simulink model "cars1"  (Simulink 7.6)
settings: Solver=ode45  StartTime=0.0  StopTime=60  RelTol=1e-3
libraries: simulink x2
settings Model: Creator=Bogdy  LastModifiedBy=Bogdy
settings OptimizationCC: BlockReduction=off  BooleanDataType=off
settings DebuggingCC: SaveWithParameterizedLinksMsg=none  SignalResolutionControl=TryResolveAllWithWarning  SolverPrmCheckMsg=none  MultiTaskDSMMsg=warning  MultiTaskCondExecSysMsg=none  StrictBusMsg=None
settings HardwareCC: TargetUnknown=on
settings RTWCC: IncludeERTFirstTime=on

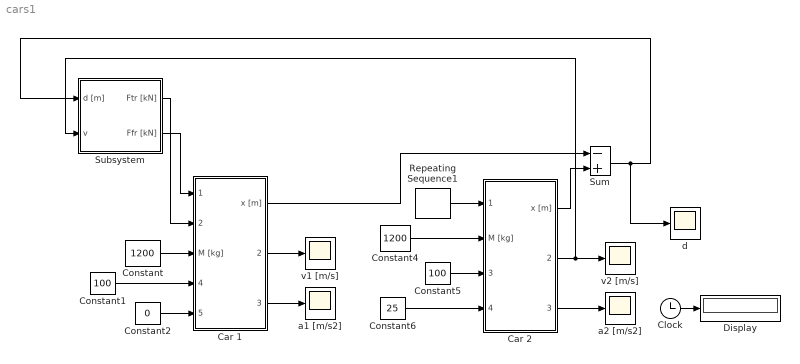
== system cars1 ==
  Car 1 : Subsystem
  Car 2 : Subsystem
  Clock : Clock
      settings: Decimation=10
  Constant : Constant  Value=1200
  Constant1 : Constant  Value=100
  Constant2 : Constant  Value=0
  Constant4 : Constant  Value=1200
  Constant5 : Constant  Value=100
  Constant6 : Constant  Value=25
  Display : Display
  Repeating Sequence1 : simulink/Sources/Repeating Sequence  SystemSampleTime=-1  rep_seq_t=[0 1 5 10 20 30 40 50 59 60]  rep_seq_y=[1 4 4 0 -2 -3 1 2 -1 1]
  Subsystem : Subsystem
  Sum : Sum  Inputs=-+  SaturateOnIntegerOverflow=on  InputSameDT=on  OutDataTypeStr=Inherit: Same as first input
  a1 [m/s2] : Scope
      settings: TimeRange=70  YMin=-4  YMax=4  SaveName=ScopeData2
  a2 [m/s2] : Scope
      settings: SaveName=ScopeData3
  d : Scope
      settings: TimeRange=60  YMin=0  YMax=550
  v1 [m/s] : Scope
  v2 [m/s] : Scope
      settings: YMin=0  YMax=550  SaveName=ScopeData4
  wires:
  Car 1/2(v [km/h]) -> v1 [m/s]/1
  Car 1/3(a [m/s2]) -> a1 [m/s2]/1
  Constant/1 -> Car 1/3(M [kg])
  Constant1/1 -> Car 1/4(V0 [km/h])
  Constant2/1 -> Car 1/5(X0 [m])
  Car 2/2(v [km/h]) -> v2 [m/s]/1, Subsystem/2(v)
  Car 2/3(a [m/s2]) -> a2 [m/s2]/1
  Constant4/1 -> Car 2/2(M [kg])
  Constant5/1 -> Car 2/3(V0 [km/h])
  Constant6/1 -> Car 2/4(X0 [m])
  Repeating Sequence1/1 -> Car 2/1(Ftr [kN])
  Sum/1 -> Subsystem/1(d [m]), d/1
  Clock/1 -> Display/1
  Subsystem/1(Ftr [kN]) -> Car 1/2(Ffr [kN])
  Subsystem/2(Ffr [kN]) -> Car 1/1(Ftr [kN])
  Car 2/1(x [m]) -> Sum/2
  Car 1/1(x [m]) -> Sum/1

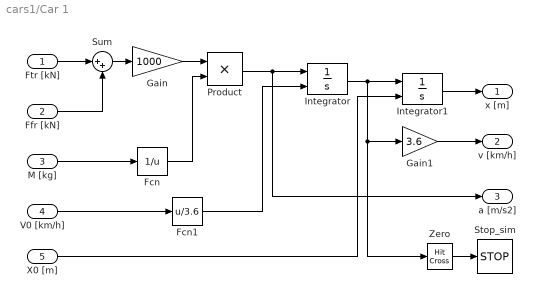
== system cars1/Car 1 ==
  Ftr [kN] : Inport
  Ffr [kN] : Inport  Port=2
  M [kg] : Inport  Port=3
  V0 [km/h] : Inport  Port=4
  X0 [m] : Inport  Port=5
  Fcn : Fcn  Expr=1/u
  Fcn1 : Fcn  Expr=u/3.6
  Gain : Gain  Gain=1000  SaturateOnIntegerOverflow=on  OutDataTypeStr=Inherit: Same as input  ParamDataTypeStr=Inherit: Same as input
  Gain1 : Gain  Gain=3.6  SaturateOnIntegerOverflow=on  OutDataTypeStr=Inherit: Same as input  ParamDataTypeStr=Inherit: Same as input
  Integrator : Integrator  InitialConditionSource=external
  Integrator1 : Integrator  InitialConditionSource=external
  Product : Product  SaturateOnIntegerOverflow=on  RndMeth=Zero  InputSameDT=on  OutDataTypeStr=Inherit: Same as first input
  Stop_sim : Stop
  Sum : Sum  Inputs=|++  SaturateOnIntegerOverflow=on  InputSameDT=on  OutDataTypeStr=Inherit: Same as first input
  Zero : HitCross  HitCrossingOffset=1  HitCrossingDirection=falling
  x [m] : Outport
  v [km/h] : Outport  Port=2
  a [m/s2] : Outport  Port=3
  wires:
  Ffr [kN]/1 -> Sum/2
  M [kg]/1 -> Fcn/1
  Sum/1 -> Gain/1
  Fcn/1 -> Product/2
  Product/1 -> Integrator/1, a [m/s2]/1
  V0 [km/h]/1 -> Fcn1/1
  Integrator/1 -> Integrator1/1, Gain1/1, Zero/1
  X0 [m]/1 -> Integrator1/2
  Integrator1/1 -> x [m]/1
  Fcn1/1 -> Integrator/2
  Gain1/1 -> v [km/h]/1
  Zero/1 -> Stop_sim/1
  Ftr [kN]/1 -> Sum/1
  Gain/1 -> Product/1

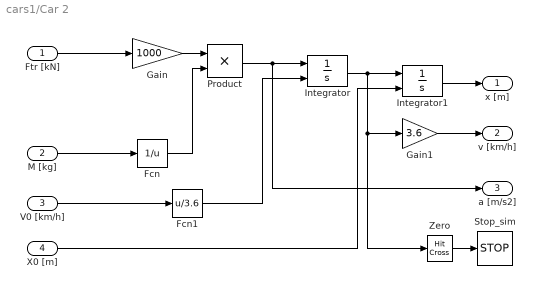
== system cars1/Car 2 ==
  Ftr [kN] : Inport
  M [kg] : Inport  Port=2
  V0 [km/h] : Inport  Port=3
  X0 [m] : Inport  Port=4
  Fcn : Fcn  Expr=1/u
  Fcn1 : Fcn  Expr=u/3.6
  Gain : Gain  Gain=1000  SaturateOnIntegerOverflow=on  OutDataTypeStr=Inherit: Same as input  ParamDataTypeStr=Inherit: Same as input
  Gain1 : Gain  Gain=3.6  SaturateOnIntegerOverflow=on  OutDataTypeStr=Inherit: Same as input  ParamDataTypeStr=Inherit: Same as input
  Integrator : Integrator  InitialConditionSource=external
  Integrator1 : Integrator  InitialConditionSource=external
  Product : Product  SaturateOnIntegerOverflow=on  RndMeth=Zero  InputSameDT=on  OutDataTypeStr=Inherit: Same as first input
  Stop_sim : Stop
  Zero : HitCross  HitCrossingOffset=1  HitCrossingDirection=falling
  x [m] : Outport
  v [km/h] : Outport  Port=2
  a [m/s2] : Outport  Port=3
  wires:
  M [kg]/1 -> Fcn/1
  Fcn/1 -> Product/2
  Product/1 -> Integrator/1, a [m/s2]/1
  V0 [km/h]/1 -> Fcn1/1
  Integrator/1 -> Integrator1/1, Gain1/1, Zero/1
  X0 [m]/1 -> Integrator1/2
  Integrator1/1 -> x [m]/1
  Fcn1/1 -> Integrator/2
  Gain1/1 -> v [km/h]/1
  Zero/1 -> Stop_sim/1
  Ftr [kN]/1 -> Gain/1
  Gain/1 -> Product/1

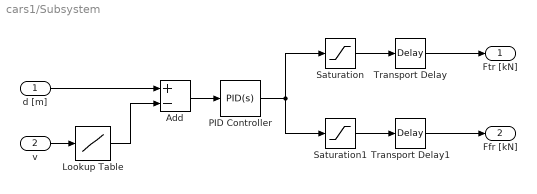
== system cars1/Subsystem ==
  d [m] : Inport
  v : Inport  Port=2
  Add : Sum  Inputs=+-
  Lookup Table : Lookup  InputValues=[5 10 25 50 100]  Table=[-1.5 -0.5 0 0.5 1.5]
  PID Controller : simulink/Continuous/PID Controller  DialogController=pidpack.PIDConfig.pidDDGCreate  DialogControllerArgs=DataTag0  SystemSampleTime=-1  Controller=PID  TimeDomain=Continuous-time  SampleTime=1  IntegratorMethod=Forward Euler  FilterMethod=Forward Euler  Form=Parallel  P=10  I=0  D=10  N=100  InitialConditionSource=internal  InitialConditionForIntegrator=0  InitialConditionForFilter=0  ExternalReset=none  LimitOutput=off  UpperSaturationLimit=inf  LowerSaturationLimit=-inf  LinearizeAsGain=off  AntiWindupMode=none  Kb=1  TrackingMode=off  Kt=1  PParamMin=[]  PParamMax=[]  IParamMin=[]  IParamMax=[]  DParamMin=[]  DParamMax=[]  NParamMin=[]  NParamMax=[]  KbParamMin=[]  KbParamMax=[]  KtParamMin=[]  KtParamMax=[]  POutMin=[]  POutMax=[]  IOutMin=[]  IOutMax=[]  DOutMin=[]  DOutMax=[]  NOutMin=[]  NOutMax=[]  KbOutMin=[]  KbOutMax=[]  KtOutMin=[]  KtOutMax=[]  IntegratorOutMin=[]  IntegratorOutMax=[]  FilterOutMin=[]  FilterOutMax=[]  SumOutMin=[]  SumOutMax=[]  SumI1OutMin=[]  SumI1OutMax=[]  SumI2OutMin=[]  SumI2OutMax=[]  SumI3OutMin=[]  SumI3OutMax=[]  SumDOutMin=[]  SumDOutMax=[]  SaturationOutMin=[]  SaturationOutMax=[]  IntegratorContinuousStateAttributes=''  IntegratorStateMustResolveToSignalObject=off  IntegratorRTWStateStorageClass=Auto  FilterContinuousStateAttributes=''  FilterStateMustResolveToSignalObject=off  FilterRTWStateStorageClass=Auto
  Saturation : Saturate  UpperLimit=4  LowerLimit=0
  Saturation1 : Saturate  UpperLimit=0  LowerLimit=-4
  Transport Delay : TransportDelay  DelayTime=0.1  InitialOutput=0.1
  Transport Delay1 : TransportDelay  DelayTime=0.5
  Ftr [kN] : Outport
  Ffr [kN] : Outport  Port=2
  wires:
  v/1 -> Lookup Table/1
  d [m]/1 -> Add/1
  Lookup Table/1 -> Add/2
  Add/1 -> PID Controller/1
  PID Controller/1 -> Saturation/1, Saturation1/1
  Saturation/1 -> Transport Delay/1
  Saturation1/1 -> Transport Delay1/1
  Transport Delay/1 -> Ftr [kN]/1
  Transport Delay1/1 -> Ffr [kN]/1
